simulink model "IonSatSimulationE"  (R2020b)
settings: Solver=ode3  StartTime=0.0  StopTime=t_sim  FixedStep=TimeStep  MaxStep=30  MinStep=.1  RelTol=1e-3
model workspace (MAT data in the model file):
  repartition_matrix = Simulink.Parameter
  repartition_matrix.DataType = 'auto'
  repartition_matrix.Complexity = 'real'
  repartition_matrix.Dimensions = [0 0]
  wheel_number = Simulink.Parameter
  wheel_number.Value = 3
  wheel_number.DataType = 'auto'
  wheel_number.Complexity = 'real'
  wheel_number.Dimensions = [1 1]
values from neighbouring files (symbols this model uses):
  Use_IGRF = 1    [Full_model_PID_MEKF_Scenario1_Monte_Carlo.m]    (also in Full_model_PID_MEKF_Scenario3_Monte_Carlo.m; Full_model_PID_UKF_Scenario1_Monte_Carlo.m; Full_model_PID_UKF_Scenario2_Monte_Carlo.m; Full_model_PID_UKF_Scenario3_Monte_Carlo.m)
  Use_IGRF_KF = 1    [Full_model_PID_MEKF_Scenario1_Monte_Carlo.m]    (also in Full_model_PID_MEKF_Scenario3_Monte_Carlo.m; Full_model_PID_UKF_Scenario1_Monte_Carlo.m; Full_model_PID_UKF_Scenario2_Monte_Carlo.m; Full_model_PID_UKF_Scenario3_Monte_Carlo.m)
undefined symbols (not defined in the file or in its folder): att, date, deg, DiscIntNeverNeededParam, IonSataero, km, m, orbit, rad, s, sat
libraries: aerolibutil x28, vrlib x20, aerolibconvert2 x13, dspmathops x13, sharedtransform x12, simulink x9, DipoleModel x3, aerolibobsolete x3, sharedutil x3, simulink_extras x2, aerolibcelestial x2, dspstat3 x1
(part 1 of 4)
settings Model: SnapshotBufferSize=100  OrderedModelArguments=off  Creator=robin  LastModifiedBy=kang Shinok
settings SolverCC: InitialStep=.5  MaxConsecutiveMinStep=2
settings DataIOCC: SaveFormat=StructureWithTime  SaveOutput=off  SignalLogging=off  DSMLogging=off  SaveTime=off
settings OptimizationCC: DefaultParameterBehavior=Inlined  UseDivisionForNetSlopeComputation=on  GainParamInheritBuiltInType=on  UseFloatMulNetSlope=on  InlineInvariantSignals=on  PassReuseOutputArgsAs=Individual arguments  ZeroExternalMemoryAtStartup=off  ZeroInternalMemoryAtStartup=off  NoFixptDivByZeroProtection=on  EfficientFloat2IntCast=on  LifeSpan=1  OptimizeBlockOrder=speed  DifferentSizesBufferReuse=on  EfficientTunableParamExpr=on
settings DebuggingCC: ParameterTunabilityLossMsg=error
settings HardwareCC: ProdBitPerInt=16  ProdBitPerPointer=8  ProdBitPerSizeT=24  ProdBitPerPtrDiffT=24  ProdLargestAtomicFloat=None  ProdWordSize=8  ProdLongLongMode=on  ProdHWDeviceType=Microchip->PIC18
settings SFSimCC: MATLABDynamicMemAlloc=off  CustomCodeUndefinedFunction=UseInterfaceOnly
settings RTWCC: Description=Embedded Coder  SystemTargetFile=ert.tlc  TemplateMakefile=ert_default_tmf  GenerateReport=on  IncludeHyperlinkInReport=on  LaunchReport=on  GenerateTraceInfo=on  GenerateTraceReport=on  GenerateTraceReportSl=on  GenerateTraceReportSf=on  GenerateTraceReportEml=on  GenerateCodeMetricsReport=on
settings CodeAppCC: ForceParamTrailComments=on  IgnoreCustomStorageClasses=off  OperatorAnnotations=on  SimulinkDataObjDesc=on  SFDataObjDesc=on  CustomSymbolStrGlobalVar=rt$N$M  CustomSymbolStrType=$N$M  CustomSymbolStrFcn=$N$M$F  CustomSymbolStrMacro=$N$M  InsertBlockDesc=on
settings ERTTargetCC: TargetLangStandard=C99 (ISO)  GenerateSampleERTMain=on  IncludeMdlTerminateFcn=off  CombineSignalStateStructs=on  SupportAbsoluteTime=off  SupportComplex=off  SupportContinuousTime=on  SupportNonInlinedSFcns=on  InlinedParameterPlacement=NonHierarchical  ERTCustomFileTemplate=example_file_process.tlc  ERTFilePackagingFormat=CompactWithDataFile

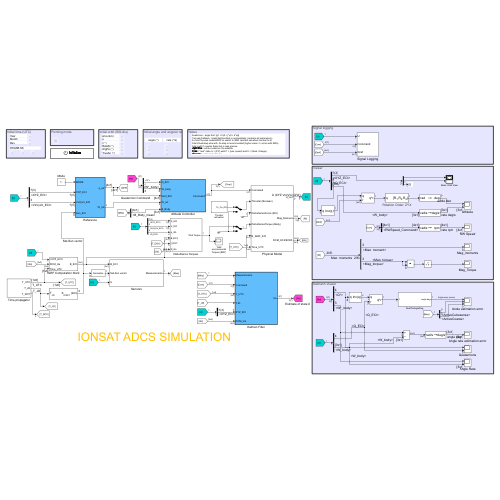
[thumbnail: Simulink's stored preview of the top-level diagram]
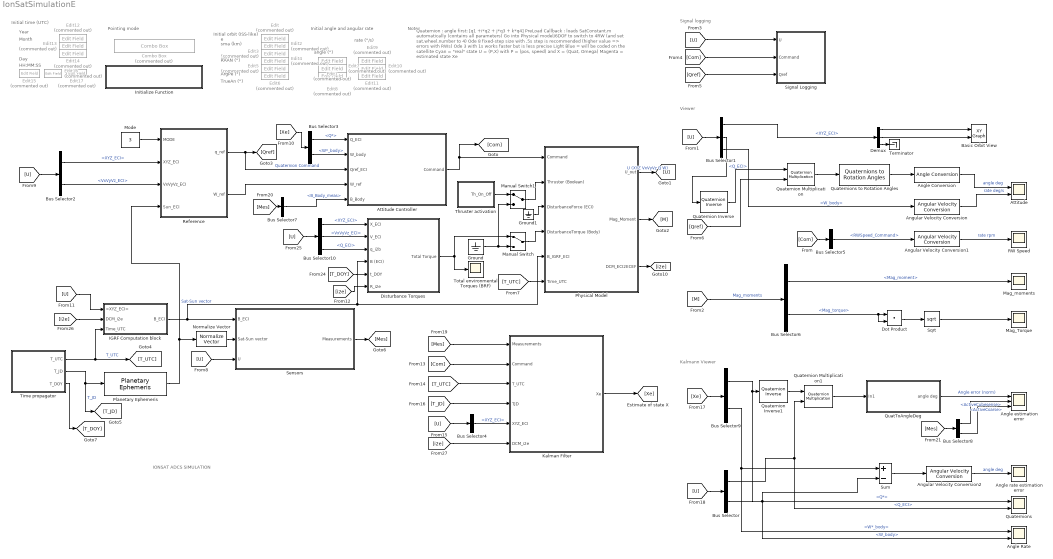
== system IonSatSimulationE ==
  note: Kalmann Viewer
  note: IONSAT ADCS SIMULATION
  note: Viewer
  note: Pointing mode
  note: Initial orbit (ISS-like)
  note: sma (km)
  note: e
  note: i (°)
  note: RAAN (°)
  note: ArgPe (°)
  note: TrueAn (°)
  note: Initial angle and angular rate
  note: angle (°)
  note: rate (°/s)
  note: Notes
  note: Quaternion : angle first: [q1 +i*q2 + j*q3 + k*q4]
      | PreLoad Callback : loads SatConstant.m automatically (contains all parameters)
      | Go into Physical model/6DOF to switch to 4RW (and set sat.wheel.number to 4)
      | Ode 8 fixed-step size with .5s step is recommended (higher value => errors with RWs)
      | Ode 3 with 1s works faster but is less precise
      | Light Blue = will be coded on the satellite
      | Cyan = "real" state U = (P,X) with P = (pos, speed) and X = (Quat, Omega)
      | Magenta = estimated state Xe
  note: Signal logging
  note: Month
  note: Year
  note: Day
  note: Initial time (UTC)
  note: HH:MM:SS
  Angle Conversion : aerolibconvert2/Angle Conversion  IU=rad  OU=deg
  Angle Rate : Scope  NumInputPorts=2
  Angle estimation error : Scope  NumInputPorts=3
  Angle rate estimation error : Scope
  Angular Velocity Conversion : aerolibconvert2/Angular Velocity Conversion  IU=rad/s  OU=deg/s
  Angular Velocity Conversion1 : aerolibconvert2/Angular Velocity Conversion  IU=rad/s  OU=rpm
  Angular Velocity Conversion2 : aerolibconvert2/Angular Velocity Conversion  IU=rad/s  OU=deg/s
  Attitude : Scope  NumInputPorts=2
  Attitude Controller : Subsystem  TreatAsAtomicUnit=on
  Basic Orbit View : simulink/Sinks/XY Graph  xmin=-1  xmax=1  ymin=-1  ymax=1  st=-1
  Bus Selector : BusSelector  OutputSignals=Q_ECI,W_body
  Bus Selector1 : BusSelector  OutputSignals=XYZ_ECI,Q_ECI,W_body
  Bus Selector10 : BusSelector  OutputSignals=XYZ_ECI,VxVyVz_ECI,Q_ECI
  Bus Selector2 : BusSelector  OutputSignals=XYZ_ECI,VxVyVz_ECI
  Bus Selector3 : BusSelector  OutputSignals=Q*,W*_body
  Bus Selector4 : BusSelector  OutputSignals=XYZ_ECI
  Bus Selector5 : BusSelector  OutputSignals=RWSpeed_Command
  Bus Selector6 : BusSelector  OutputSignals=Mag_moment,Mag_torque
  Bus Selector7 : BusSelector  OutputSignals=B_Body_meas
  Bus Selector8 : BusSelector  OutputSignals=ActiveCubesense,ActiveCoarse
  Bus Selector9 : BusSelector  OutputSignals=Q*,W*_body
  Combo Box : ComboBox  Commented=on  LabelPosition=Hide  SelectedLabel=Sun
      settings: Values={{'Nadir', 'Retrograde', 'Drag', 'Sun', 'Sun Aero', 'B-dot', 'Custom Quaternion'}, [1 5 4 3 2 6 7]}
  Demux : Demux  Outputs=3
  Disturbance Torques : Subsystem
  Dot Product : DotProduct  InputSameDT=on  OutDataTypeStr=Inherit: Inherit via internal rule
  Edit{,1..17} (18 alike) : EditField  Commented=on  LabelPosition=Hide  ShowInitialText=on  Alignment=Center
  Ground : Ground
  Ground1 : Ground
  IGRF Computation block : Subsystem
  Initialize Function : Subsystem  TreatAsAtomicUnit=on
  Kalman Filter : Subsystem  TreatAsAtomicUnit=on  SystemSampleTime=1
  Mag_Torque : Scope
  Mag_moments : Scope
  Manual Switch : ManualSwitch
  Manual Switch1 : ManualSwitch
  Mode : Constant  Value=3  OutDataTypeStr=int8
  Normalize Vector : vrlib/Utilities/Normalize Vector  maxzero=0
  Physical Model : Subsystem
      settings: MinAlgLoopOccurrences=on
  Planetary Ephemeris : aerolibcelestial/Planetary Ephemeris  kmflag=km,km/s  epochflag=Julian date  de=DE405  nCenter=Earth  nTarget=Sun  errorflag=Error  velflag=off
      settings: SourceProductBaseCode=AE
  QuatToAngleDeg : Subsystem
  Quaternion Inverse : aerolibutil/Quaternion Inverse
  Quaternion Inverse1 : aerolibutil/Quaternion Inverse
  Quaternion Multiplication : aerolibutil/Quaternion Multiplication
  Quaternion Multiplication1 : aerolibutil/Quaternion Multiplication
  Quaternions : Scope  NumInputPorts=2
  Quaternions to Rotation Angles : sharedtransform/Quaternions to Rotation Angles  rotationOrder=ZYX  aMode=aMode
      settings: SourceProductBaseCode=AE,PW,DR,MT,UV,VE
  RW Speed : Scope
  Reference : Subsystem  TreatAsAtomicUnit=on
  Sensors : Subsystem
  Signal Logging : Subsystem
  Sqrt : Sqrt  SaturateOnIntegerOverflow=on
  Sum : Sum  Inputs=+-
  Terminator : Terminator
  Thruster activation : Subsystem
  Time propagator : Subsystem
  Total environmental Torques (BRF) : Scope
  wires:
  Reference/1(q_ref) -> Attitude Controller/3(Qref_ECI), [Qref]  "Quaternion Command"
  Mode/1 -> Reference/1(MODE)
  Bus Selector2/2 -> Reference/3(VxVyVz_ECI)  "<VxVyVz_ECI>"
  Physical Model/1(U_out) -> [U]  "U (XYZ VxVyVz Q W)"
  Attitude Controller/1(Command) -> Physical Model/1(Command), [Com]
  Angle Conversion/1 -> Attitude/1  "angle deg"
  Demux/3 -> Terminator/1
  Demux/2 -> Basic Orbit View/2
  Angular Velocity Conversion/1 -> Attitude/2  "rate deg/s"
  Bus Selector1/1 -> Demux/1  "<XYZ_ECI>"
  Quaternion Multiplication/1 -> Quaternions to Rotation Angles/1
  Demux/1 -> Basic Orbit View/1
  Bus Selector1/3 -> Angular Velocity Conversion/1  "<W_body>"
  Quaternions to Rotation Angles/1 -> Angle Conversion/1
  Angular Velocity Conversion1/1 -> RW Speed/1  "rate rpm"
  [Com] -> Bus Selector5/1
  [U] -> Bus Selector1/1
  Bus Selector2/1 -> Reference/2(XYZ_ECI)  "<XYZ_ECI>"
  Bus Selector3/2 -> Attitude Controller/2(W_body)  "<W*_body>"
  Planetary Ephemeris/1 -> Reference/4(Sun_ECI), Normalize Vector/1  "Sat-Sun vector"
  [U] -> Signal Logging/1(U)
  [Com] -> Signal Logging/2(Command)
  [Qref] -> Signal Logging/3(Qref)
  [Qref] -> Quaternion Multiplication/2
  Quaternion Inverse/1 -> Quaternion Multiplication/1
  Bus Selector1/2 -> Quaternion Inverse/1  "<Q_ECI>"
  Physical Model/2(Mag_Moment) -> [M]
  [M] -> Bus Selector6/1  "Mag_moments"
  Time propagator/1(T_UTC) -> IGRF Computation block/3("Time_UTC "), [T_UTC]  "T_UTC"
  Time propagator/2(T_JD) -> [T_JD], Planetary Ephemeris/1  "T_JD"
  [U] -> Bus Selector2/1
  [Xe] -> Bus Selector3/1
  [U] -> IGRF Computation block/1(<XYZ_ECI>)
  Kalman Filter/1(Xe) -> [Xe]
  [Com] -> Kalman Filter/2(Command)
  [T_UTC] -> Kalman Filter/3(T_UTC)
  [U] -> Bus Selector4/1
  Bus Selector4/1 -> Kalman Filter/5(XYZ_ECI)  "<XYZ_ECI>"
  [T_JD] -> Kalman Filter/4(TJD)
  [Xe] -> Bus Selector9/1
  [U] -> Bus Selector/1
  Bus Selector9/2 -> Angle Rate/1, Sum/1  "<W*_body>"
  Bus Selector/2 -> Sum/2, Angle Rate/2  "<W_body>"
  Sum/1 -> Angular Velocity Conversion2/1
  Bus Selector9/1 -> Quaternions/1, Quaternion Inverse1/1  "<Q*>"
  Quaternion Inverse1/1 -> Quaternion Multiplication1/1
  Bus Selector/1 -> Quaternions/2, Quaternion Multiplication1/2  "<Q_ECI>"
  Angular Velocity Conversion2/1 -> Angle rate estimation error/1  "angle deg"
  Bus Selector5/1 -> Angular Velocity Conversion1/1  "<RWSpeed_Command>"
  Bus Selector6/1 -> Mag_moments/1  "<Mag_moment>"
  Bus Selector6/2 -> Dot Product/2, Dot Product/1  "<Mag_torque>"
  Dot Product/1 -> Sqrt/1
  Sqrt/1 -> Mag_Torque/1
  Bus Selector7/1 -> Attitude Controller/5(B_Body)  "<B_Body_meas>"
  [U] -> Sensors/3(U)
  Sensors/1(Measurements) -> [Mes]
  [Mes] -> Kalman Filter/1(Measurements)
  [Mes] -> Bus Selector7/1
  [Mes] -> Bus Selector8/1
  Bus Selector8/1 -> Angle estimation error/2  "<ActiveCubesense>"
  Bus Selector8/2 -> Angle estimation error/3  "<ActiveCoarse>"
  Quaternion Multiplication1/1 -> QuatToAngleDeg/1(In1)
  QuatToAngleDeg/1(angle deg) -> Angle estimation error/1  "Angle error (norm)"
  [U] -> Bus Selector10/1
  Bus Selector10/3 -> Disturbance Torques/3(q_i2b)  "<Q_ECI>"
  Bus Selector10/1 -> Disturbance Torques/1(X_ECI)  "<XYZ_ECI>"
  Bus Selector3/1 -> Attitude Controller/1(Q_ECI)  "<Q*>"
  Bus Selector10/2 -> Disturbance Torques/2(V_ECI)  "<VxVyVz_ECI>"
  Time propagator/3(T_DOY) -> [T_DOY]
  [T_DOY] -> Disturbance Torques/5(t_DOY)
  [i2e] -> IGRF Computation block/2("DCM_i2e ")
  IGRF Computation block/1(B_ECI) -> Sensors/1(B_ECI), Physical Model/5(B_IGRF_ECI), Disturbance Torques/4(B (ECI))
  [i2e] -> Kalman Filter/6("DCM_i2e ")
  Normalize Vector/1 -> Sensors/2(Sat-Sun vector)
  [i2e] -> Disturbance Torques/6(R_i2e)
  Ground/1 -> Manual Switch/2, Manual Switch1/2
  Manual Switch1/1 -> Physical Model/2(Thruster (Boolean))
  Thruster activation/1(Th_On_Off) -> Manual Switch1/1
  Disturbance Torques/1("Total Torque ") -> Manual Switch/1, Total environmental Torques (BRF)/1
  Manual Switch/1 -> Physical Model/4(DisturbanceTorque (Body))
  [T_UTC] -> Physical Model/6(Time_UTC)
  Physical Model/3(DCM_ECI2ECEF) -> [i2e]
  Ground1/1 -> Physical Model/3(DisturbanceForce (ECI))
  Reference/2(W_ref) -> Attitude Controller/4(W_ref)

== system IonSatSimulationE/Attitude Controller ==
  note: Choix d'un contrôleur PID : plus simple et robuste qu'un LQR/SliddingSurface ou autre
  note: Runs as fast as possible
  note: Runs at 1Hz
  Q_ECI : Inport
  W_body : Inport  Port=2
  Qref_ECI : Inport  Port=3
  W_ref : Inport  Port=4
  B_Body : Inport  Port=5
  Abs : Abs
  B-dot choice1 : Subsystem
  B-dot choice2 : Subsystem
  B-dot command : Subsystem  TreatAsAtomicUnit=on
  Bus Creator : BusCreator  Inputs=2
  Constant : Constant
  Constant1 : Constant  Value=0
  Ground2 : Ground  Commented=on
  If : If  IfExpression=u1 > 0.068
  If Action Subsystem : Subsystem  TreatAsAtomicUnit=on
  If Action Subsystem1 : Subsystem  TreatAsAtomicUnit=on
  Max of Elements : MinMax  Function=max
  Merge : Merge
  PID (nominal command) : Subsystem  TreatAsAtomicUnit=on  SystemSampleTime=1
  RW4 : Subsystem  Commented=on
  Scope : Scope
  Scope1 : Scope
  Command : Outport  VectorParamsAs1DForOutWhenUnconnected=off
  wires:
  Ground2/1 -> RW4/1(Mc (scalar))
  B_Body/1 -> PID (nominal command)/4(B_IGRF_Body), B-dot command/1(B)
  B-dot choice2/1(output command) -> Bus Creator/2  "Magnetotorquer_Command"
  B-dot choice1/1(output command) -> Bus Creator/1  "RWSpeed_Command"
  B-dot command/2(Wheel command (0)) -> B-dot choice1/2(Command (B-dot))
  B-dot command/1(Magnetic moment (B-dot)) -> B-dot choice2/2(Command (B-dot))
  Q_ECI/1 -> PID (nominal command)/1(Q_ECI)
  Qref_ECI/1 -> PID (nominal command)/2(Qref_ECI)
  PID (nominal command)/1(RW Command) -> B-dot choice1/1(" command (normal)")
  PID (nominal command)/2(Mag Command) -> B-dot choice2/1(" command (normal)")
  Bus Creator/1 -> Command/1
  Abs/1 -> Max of Elements/1
  If/1 -> If Action Subsystem/Action
  If Action Subsystem1/1(Out1) -> Merge/2
  Max of Elements/1 -> Scope1/1, If/1
  If/2 -> If Action Subsystem1/Action
  If Action Subsystem/1(Out1) -> Merge/1
  Constant/1 -> If Action Subsystem/1(In1)
  Merge/1 -> PID (nominal command)/6(No wheels use), Scope/1, B-dot choice2/3(B_dot mode (0/1)), B-dot choice1/3(B_dot mode (0/1))
  Constant1/1 -> If Action Subsystem1/1(In1)
  W_body/1 -> PID (nominal command)/3(W_Body), Abs/1
  W_ref/1 -> PID (nominal command)/5(W_ref)

== system IonSatSimulationE/Disturbance Torques ==
  X_ECI : Inport
  V_ECI : Inport  Port=2
  q_i2b : Inport  Port=3
  B (ECI) : Inport  Port=4
  t_DOY : Inport  Port=5
  R_i2e : Inport  Port=6
  3 dist torques : Scope  NumInputPorts=3
  Add1 : Sum  Inputs=+++
  Aerodynamic Model : Subsystem
  Gravity Gradient Model : Subsystem
  Ground : Ground
  Ground1 : Ground
  Ground2 : Ground
  Magnetic Torque Model : Subsystem
  Manual Switch : ManualSwitch
  Manual Switch1 : ManualSwitch
  Manual Switch2 : ManualSwitch
  Quaternions to Direction Cosine Matrix : sharedtransform/Quaternions to  Direction Cosine Matrix  aMode=aMode
      settings: SourceProductBaseCode=AE,PW,DR,MT,UV,VE
  Total Torque : Scope
  "Total Torque " : Outport
  wires:
  Add1/1 -> Total Torque/1, "Total Torque "/1
  V_ECI/1 -> Aerodynamic Model/1(Velocity  (V) [m/s])
  X_ECI/1 -> Aerodynamic Model/2(Position (X) [m]), Gravity Gradient Model/1("Position (X) [m] ")
  Manual Switch/1 -> 3 dist torques/1, Add1/1  "Aero Torque"
  Manual Switch2/1 -> Add1/3, 3 dist torques/3  "GG Torque"
  B (ECI)/1 -> Magnetic Torque Model/1(B (ECI))
  Manual Switch1/1 -> Add1/2, 3 dist torques/2  "Magnetic Torque"
  q_i2b/1 -> Quaternions to Direction Cosine Matrix/1
  Quaternions to Direction Cosine Matrix/1 -> Gravity Gradient Model/2(Attitude (DCMi2b)), Magnetic Torque Model/2(Attitude (DCMi2b)), Aerodynamic Model/3(Attitude (DCM_i2b))  "i2b"
  R_i2e/1 -> Aerodynamic Model/5(DCM_i2e)
  t_DOY/1 -> Aerodynamic Model/4(DOY)
  Ground/1 -> Manual Switch/2
  Aerodynamic Model/1(Aero. Torque [N.m]) -> Manual Switch/1  "Aero Torque"
  Magnetic Torque Model/1(MagneticTorque (N.m)) -> Manual Switch1/1  "Magnetic Torque"
  Ground1/1 -> Manual Switch1/2
  Ground2/1 -> Manual Switch2/2
  Gravity Gradient Model/1(Gravity Gradient [N.m]) -> Manual Switch2/1  "GG Torque"

== system IonSatSimulationE/IGRF Computation block ==
  <XYZ_ECI> : Inport
  "DCM_i2e " : Inport  Port=2
  "Time_UTC " : Inport  Port=3
  Bus Creator : BusCreator  Inputs=5
  Bus Selector4 : BusSelector  OutputSignals=XYZ_ECI
  Demux : Demux  Outputs=2
  ECI To LLA : MATLAB Function  TreatAsAtomicUnit=on
  Obtain B_ECI : Subsystem
  Product : Product  Multiplication=Matrix(*)
  Reshape : Reshape  OutputDimensionality=Row vector (2-D)
  Terminator : Terminator
  B_ECI : Outport  VectorParamsAs1DForOutWhenUnconnected=off
  wires:
  ECI To LLA/3(long) -> Bus Creator/3
  ECI To LLA/2(lat) -> Bus Creator/2
  ECI To LLA/1(h) -> Bus Creator/1
  Demux/1 -> Bus Creator/4
  Demux/2 -> Terminator/1
  "DCM_i2e "/1 -> Product/2, Bus Creator/5  "DCM_i2e"
  <XYZ_ECI>/1 -> Bus Selector4/1
  Reshape/1 -> Product/1
  Product/1 -> ECI To LLA/1(X_ECEF)
  Bus Selector4/1 -> Reshape/1  "<XYZ_ECI>"
  Bus Creator/1 -> Obtain B_ECI/1(In1)
  Obtain B_ECI/1(Out1) -> B_ECI/1
  "Time_UTC "/1 -> Demux/1

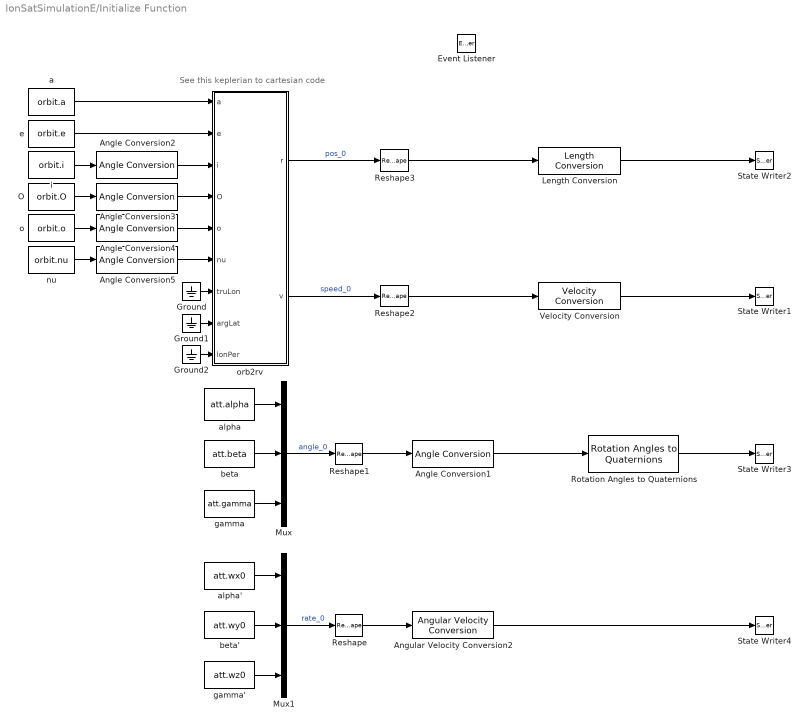
== system IonSatSimulationE/Initialize Function ==
  note: See this keplerian to cartesian code
  Angle Conversion{1..5} (5 alike) : aerolibconvert2/Angle Conversion  IU=deg  OU=rad
  Angular Velocity Conversion2 : aerolibconvert2/Angular Velocity Conversion  IU=deg/s  OU=rad/s
  Event Listener : EventListener  DisableCoverage=on  EventName=reset
  Ground : Ground
  Ground1 : Ground
  Ground2 : Ground
  Length Conversion : aerolibconvert2/Length Conversion  IU=km  OU=m
  Mux : Mux  Inputs=3
  Mux1 : Mux  Inputs=3
  O : Constant  Value=orbit.O
  Reshape{,1..3} (4 alike) : Reshape  OutputDimensionality=Column vector (2-D)
  Rotation Angles to Quaternions : sharedtransform/Rotation Angles to Quaternions  rotationOrder=ZYX  aMode=aMode
      settings: SourceProductBaseCode=AE,PW,DR,MT,UV,VE
  State Writer1 : StateWriter  StateOwnerBlock=../../Physical Model/6DOF in ECI frame/Integrator_speed
  State Writer2 : StateWriter  StateOwnerBlock=../../Physical Model/6DOF in ECI frame/Integrator_pos
  State Writer3 : StateWriter  StateOwnerBlock=../../Physical Model/6DOF in ECI frame/Compute Q_ECI/Integrator_quat
  State Writer4 : StateWriter  StateOwnerBlock=../../Physical Model/6DOF in ECI frame/Integrator_rate
  Velocity Conversion : aerolibconvert2/Velocity Conversion  IU=km/s  OU=m/s
  a : Constant  Value=orbit.a
  alpha : Constant  Value=att.alpha
  alpha' : Constant  Value=att.wx0
  beta : Constant  Value=att.beta
  beta' : Constant  Value=att.wy0
  e : Constant  Value=orbit.e
  gamma : Constant  Value=att.gamma
  gamma' : Constant  Value=att.wz0
  i : Constant  Value=orbit.i
  nu : Constant  Value=orbit.nu
  o : Constant  Value=orbit.o
  orb2rv : MATLAB Function  TreatAsAtomicUnit=on
  wires:
  Angular Velocity Conversion2/1 -> State Writer4/1
  Angle Conversion1/1 -> Rotation Angles to Quaternions/1
  orb2rv/1(r) -> Reshape3/1  "pos_0"
  Mux1/1 -> Reshape/1  "rate_0"
  Mux/1 -> Reshape1/1  "angle_0"
  orb2rv/2(v) -> Reshape2/1  "speed_0"
  Rotation Angles to Quaternions/1 -> State Writer3/1
  Reshape/1 -> Angular Velocity Conversion2/1
  Reshape1/1 -> Angle Conversion1/1
  Reshape2/1 -> Velocity Conversion/1
  Reshape3/1 -> Length Conversion/1
  a/1 -> orb2rv/1(a)
  e/1 -> orb2rv/2(e)
  i/1 -> Angle Conversion2/1
  O/1 -> Angle Conversion3/1
  o/1 -> Angle Conversion4/1
  nu/1 -> Angle Conversion5/1
  Angle Conversion2/1 -> orb2rv/3(i)
  Angle Conversion3/1 -> orb2rv/4(O)
  Angle Conversion4/1 -> orb2rv/5(o)
  Angle Conversion5/1 -> orb2rv/6(nu)
  Ground/1 -> orb2rv/7(truLon)
  Ground1/1 -> orb2rv/8(argLat)
  Ground2/1 -> orb2rv/9(lonPer)
  Length Conversion/1 -> State Writer2/1
  Velocity Conversion/1 -> State Writer1/1
  alpha/1 -> Mux/1
  beta/1 -> Mux/2
  gamma/1 -> Mux/3
  alpha'/1 -> Mux1/1
  gamma'/1 -> Mux1/3
  beta'/1 -> Mux1/2

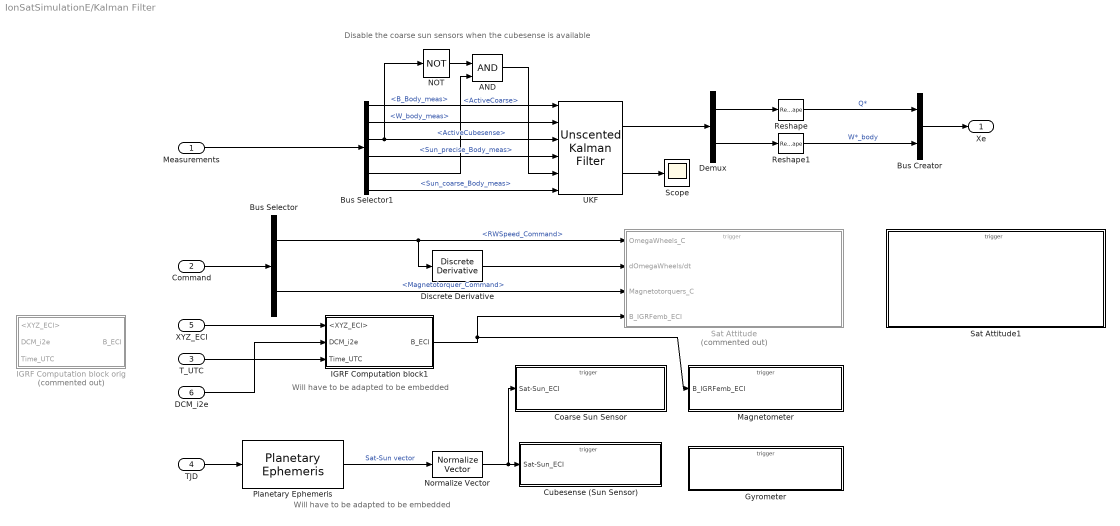
== system IonSatSimulationE/Kalman Filter ==
  note: Disable the coarse sun sensors when the cubesense is available
  note: Will have to be adapted to be embedded
  note: Will have to be adapted to be embedded
  Measurements : Inport
  Command : Inport  Port=2
  T_UTC : Inport  Port=3
  TJD : Inport  Port=4
  XYZ_ECI : Inport  Port=5
  "DCM_i2e " : Inport  Port=6
  AND : Logic  IconShape=distinctive  AllPortsSameDT=off  OutDataTypeStr=boolean
  Bus Creator : BusCreator  Inputs=2
  Bus Selector : BusSelector  OutputSignals=RWSpeed_Command,Magnetotorquer_Command
  Bus Selector1 : BusSelector  OutputSignals=B_Body_meas,W_body_meas,ActiveCubesense,Sun_precise_Body_meas,ActiveCoarse,Sun_coarse_Body_meas
  Coarse Sun Sensor : Subsystem  TreatAsAtomicUnit=on
  Cubesense (Sun Sensor) : Subsystem  TreatAsAtomicUnit=on
  Demux : Demux  Outputs=2
  Discrete Derivative : simulink/Discrete/Discrete Derivative  gainval=1.0  ICPrevScaledInput=0.0  OutMin=[]  OutMax=[]  OutDataType=fixdt(1, 16)  OutScaling=2^-10  DoSatur=off
  Gyrometer : Subsystem  TreatAsAtomicUnit=on
  IGRF Computation block orig : Subsystem  Commented=on
  IGRF Computation block1 : Subsystem
  Magnetometer : Subsystem  TreatAsAtomicUnit=on
  NOT : Logic  Operator=NOT  IconShape=distinctive  AllPortsSameDT=off  OutDataTypeStr=boolean
  Normalize Vector : vrlib/Utilities/Normalize Vector  maxzero=0
  Planetary Ephemeris : aerolibcelestial/Planetary Ephemeris  kmflag=km,km/s  epochflag=Julian date  de=DE405  nCenter=Earth  nTarget=Sun  errorflag=Error  velflag=off
      settings: SourceProductBaseCode=AE
  Reshape : Reshape  OutputDimensionality=Customize  OutputDimensions=[4]
  Reshape1 : Reshape  OutputDimensionality=Customize  OutputDimensions=[3]
  Sat Attitude : Subsystem  Commented=on  TreatAsAtomicUnit=on
  Sat Attitude1 : Subsystem  TreatAsAtomicUnit=on
  Scope : Scope
  UKF : sharedTrackingLibrary/Unscented Kalman Filter  StateTransitionFcn=SatAttitude  HasAdditiveProcessNoise=Additive  ProcessNoise=5e-7  HasTimeVaryingProcessNoise=off  HasStateTransitionFcnExtraArgument=0  InitialState=[1 0 0 0 0 0 0]  InitialStateCovariance=1e-7  Alpha=8e-2  Beta=2  Kappa=0  MeasurementFcn1=MagMeasure  HasMeasurementEnablePort1=off  HasAdditiveMeasurementNoise1=Additive  MeasurementNoise1=sat.sensors.mag_sigma*sat.sensors.mag_sigma*ones(3,1)  HasTimeVaryingMeasurementNoise1=off  HasMeasurementFcnExtraArgument1=0  MeasurementFcn2=GyroMeasure  HasMeasurementEnablePort2=off  HasAdditiveMeasurementNoise2=Additive  MeasurementNoise2=sat.sensors.gyro_sigma*sat.sensors.gyro_sigma*ones(3,1)  HasTimeVaryingMeasurementNoise2=off  HasMeasurementFcnExtraArgument2=0  MeasurementFcn3=SunMeasure  HasMeasurementEnablePort3=on  HasAdditiveMeasurementNoise3=Additive  MeasurementNoise3=sat.sensors.sun_sigma*sat.sensors.sun_sigma*ones(3,1)  HasTimeVaryingMeasurementNoise3=off  HasMeasurementFcnExtraArgument3=0  MeasurementFcn4=SunMeasureCoarse  HasMeasurementEnablePort4=on  HasAdditiveMeasurementNoise4=Additive  MeasurementNoise4=sat.sensors.sun_coarse_sigma*sat.sensors.sun_coarse_sigma*ones(3,1)  HasTimeVaryingMeasurementNoise4=off  HasMeasurementFcnExtraArgument4=0  MeasurementFcn5=myMeasurementFcn  HasMeasurementEnablePort5=off  HasAdditiveMeasurementNoise5=Additive  MeasurementNoise5=1  HasTimeVaryingMeasurementNoise5=off  HasMeasurementFcnExtraArgument5=0  EnableMultirate=off  StateTransitionFcnSampleTime=1  MeasurementFcn1SampleTime=1  MeasurementFcn2SampleTime=1  MeasurementFcn3SampleTime=1  MeasurementFcn4SampleTime=1  MeasurementFcn5SampleTime=1  UseCurrentEstimator=on  OutputStateCovariance=on  DataType=double  SampleTime=1  NumberOfMeasurements=4
      settings: SourceProductBaseCode=AE,PW,CT,DR,TF,ID,LP,NV,AR,RO,RR,UV,VE
  Xe : Outport  VectorParamsAs1DForOutWhenUnconnected=off
  wires:
  Measurements/1 -> Bus Selector1/1
  UKF/1 -> Demux/1
  XYZ_ECI/1 -> IGRF Computation block1/1(<XYZ_ECI>)
  T_UTC/1 -> IGRF Computation block1/3("Time_UTC ")
  IGRF Computation block1/1(B_ECI) -> Sat Attitude/4(B_IGRFemb_ECI), Magnetometer/1(B_IGRFemb_ECI)
  Command/1 -> Bus Selector/1
  Bus Selector/1 -> Discrete Derivative/1, Sat Attitude/1(OmegaWheels_C)  "<RWSpeed_Command>"
  Bus Selector/2 -> Sat Attitude/3(Magnetotorquers_C)  "<Magnetotorquer_Command>"
  TJD/1 -> Planetary Ephemeris/1
  Bus Selector1/1 -> UKF/1  "<B_Body_meas>"
  Bus Selector1/2 -> UKF/2  "<W_body_meas>"
  Bus Selector1/6 -> UKF/6  "<Sun_coarse_Body_meas>"
  Planetary Ephemeris/1 -> Normalize Vector/1  "Sat-Sun vector"
  Discrete Derivative/1 -> Sat Attitude/2(dOmegaWheels/dt)
  Bus Selector1/3 -> UKF/3, NOT/1  "<ActiveCubesense>"
  Bus Selector1/4 -> UKF/4  "<Sun_precise_Body_meas>"
  Bus Selector1/5 -> AND/2  "<ActiveCoarse>"
  NOT/1 -> AND/1
  AND/1 -> UKF/5
  UKF/2 -> Scope/1
  Bus Creator/1 -> Xe/1
  Demux/1 -> Reshape/1
  Demux/2 -> Reshape1/1
  Reshape/1 -> Bus Creator/1  "Q*"
  Reshape1/1 -> Bus Creator/2  "W*_body"
  "DCM_i2e "/1 -> IGRF Computation block1/2("DCM_i2e ")
  Normalize Vector/1 -> Coarse Sun Sensor/1(Sat-Sun_ECI), Cubesense (Sun Sensor)/1(Sat-Sun_ECI)

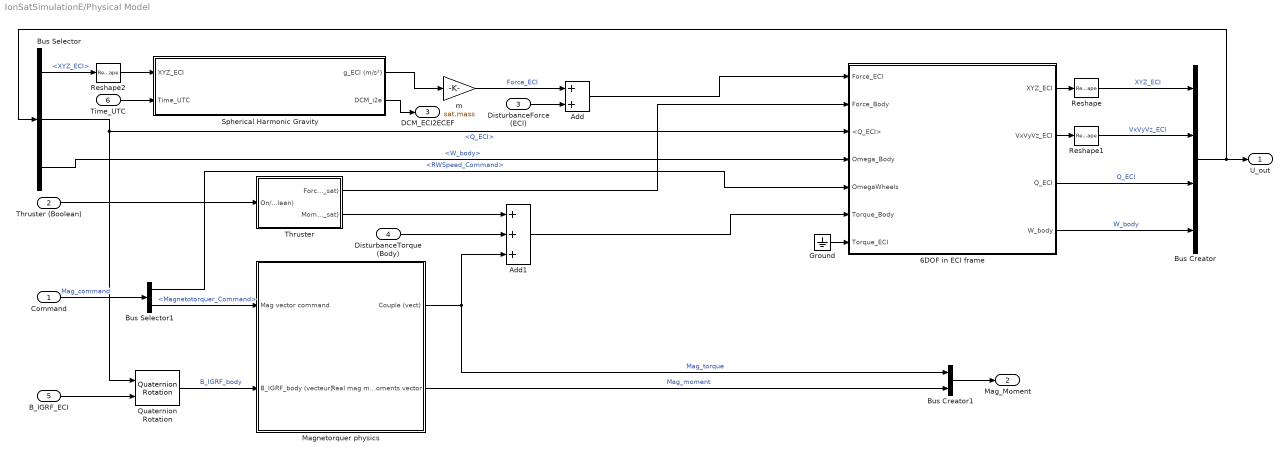
== system IonSatSimulationE/Physical Model ==
  Command : Inport
  Thruster (Boolean) : Inport  Port=2
  DisturbanceForce (ECI) : Inport  Port=3
  DisturbanceTorque (Body) : Inport  Port=4
  B_IGRF_ECI : Inport  Port=5
  Time_UTC : Inport  Port=6
  6DOF in ECI frame : Subsystem
  Add : Sum
  Add1 : Sum  Inputs=+++
  Bus Creator : BusCreator  Inputs=4
  Bus Creator1 : BusCreator  Inputs=2
  Bus Selector : BusSelector  OutputSignals=XYZ_ECI,Q_ECI,W_body
  Bus Selector1 : BusSelector  OutputSignals=RWSpeed_Command,Magnetotorquer_Command
  Ground : Ground
  Magnetorquer physics : Subsystem
  Quaternion Rotation : aerolibutil/Quaternion Rotation
  Reshape : Reshape
  Reshape1 : Reshape
  Reshape2 : Reshape  OutputDimensionality=Column vector (2-D)
  Spherical Harmonic Gravity : Subsystem  TreatAsAtomicUnit=on  SystemSampleTime=1
  Thruster : Subsystem
  m : Gain  Gain=sat.mass
  U_out : Outport  VectorParamsAs1DForOutWhenUnconnected=off
  Mag_Moment : Outport  Port=2  VectorParamsAs1DForOutWhenUnconnected=off
  DCM_ECI2ECEF : Outport  Port=3
  wires:
  Bus Selector/1 -> Reshape2/1  "<XYZ_ECI>"
  Spherical Harmonic Gravity/1(g_ECI (m/s²)) -> m/1
  Thruster (Boolean)/1 -> Thruster/1(On/Off (Boolean))
  Bus Creator/1 -> Bus Selector/1, U_out/1
  Bus Selector/2 -> 6DOF in ECI frame/3(<Q_ECI>), Quaternion Rotation/1  "<Q_ECI>"
  6DOF in ECI frame/3(Q_ECI) -> Bus Creator/3  "Q_ECI"
  6DOF in ECI frame/1(XYZ_ECI) -> Reshape/1
  6DOF in ECI frame/2(VxVyVz_ECI) -> Reshape1/1
  m/1 -> Add/1  "Force_ECI"
  Add/1 -> 6DOF in ECI frame/1(Force_ECI)
  Thruster/1(Force (G_sat)) -> 6DOF in ECI frame/2(Force_Body)
  Bus Selector1/2 -> Magnetorquer physics/1(Mag vector command)  "<Magnetotorquer_Command>"
  Thruster/2(Moment (G_sat)) -> Add1/1
  Add1/1 -> 6DOF in ECI frame/6(Torque_Body)
  DisturbanceForce (ECI)/1 -> Add/2
  DisturbanceTorque (Body)/1 -> Add1/2
  Reshape/1 -> Bus Creator/1  "XYZ_ECI"
  Reshape1/1 -> Bus Creator/2  "VxVyVz_ECI"
  Reshape2/1 -> Spherical Harmonic Gravity/1(XYZ_ECI)
  Bus Selector/3 -> 6DOF in ECI frame/4("Omega_Body ")  "<W_body>"
  Time_UTC/1 -> Spherical Harmonic Gravity/2(Time_UTC)
  B_IGRF_ECI/1 -> Quaternion Rotation/2
  Quaternion Rotation/1 -> Magnetorquer physics/2(B_IGRF_body (vecteur))  "B_IGRF_body"
  Magnetorquer physics/2(Real mag moments vector) -> Bus Creator1/2  "Mag_moment"
  Magnetorquer physics/1(Couple (vect)) -> Add1/3, Bus Creator1/1  "Mag_torque"
  6DOF in ECI frame/4(W_body) -> Bus Creator/4  "W_body"
  Command/1 -> Bus Selector1/1  "Mag_command"
  Bus Selector1/1 -> 6DOF in ECI frame/5(OmegaWheels)  "<RWSpeed_Command>"
  Bus Creator1/1 -> Mag_Moment/1
  Spherical Harmonic Gravity/2(DCM_i2e) -> DCM_ECI2ECEF/1
  Ground/1 -> 6DOF in ECI frame/7(Torque_ECI)

== system IonSatSimulationE/QuatToAngleDeg ==
  In1 : Inport
  Abs : Abs
  Angle Conversion1 : aerolibconvert2/Angle Conversion  IU=rad  OU=deg
  Demux1 : Demux
  Quaternion to axis and angle conversion : MATLABFcn  MATLABFcn=quat2axisangle
  Terminator1 : Terminator
  Terminator2 : Terminator
  Terminator3 : Terminator
  angle deg : Outport  VectorParamsAs1DForOutWhenUnconnected=off
  wires:
  Demux1/2 -> Terminator2/1
  Demux1/4 -> Angle Conversion1/1
  In1/1 -> Quaternion to axis and angle conversion/1
  Demux1/1 -> Terminator1/1
  Demux1/3 -> Terminator3/1
  Quaternion to axis and angle conversion/1 -> Demux1/1
  Abs/1 -> angle deg/1
  Angle Conversion1/1 -> Abs/1  "angle deg"

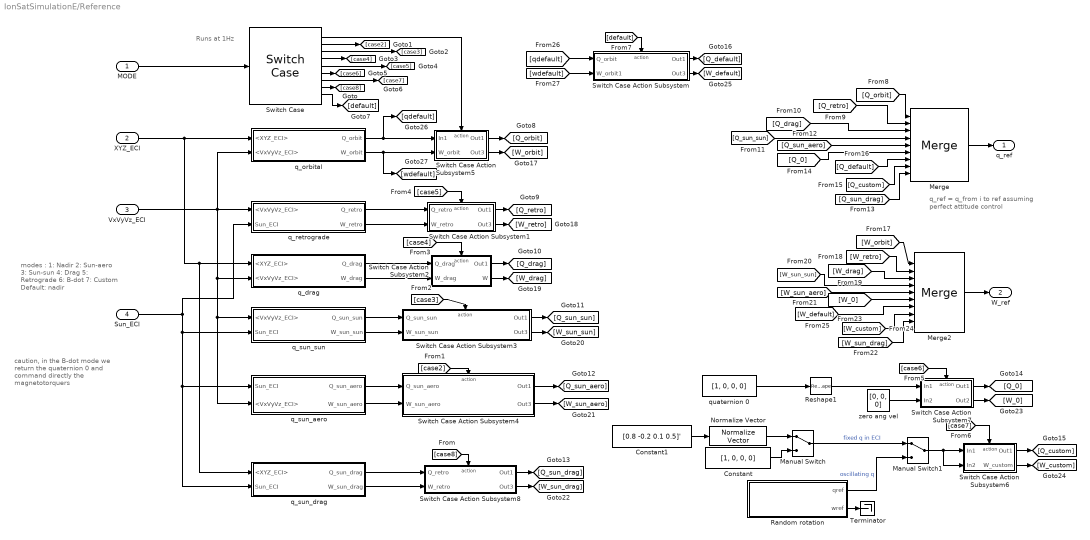
== system IonSatSimulationE/Reference ==
  note: caution, in the B-dot mode we return the quaternion 0 and command directly the magnetotorquers
  note: modes :
      | 1: Nadir
      | 2: Sun-aero
      | 3: Sun-sun
      | 4: Drag
      | 5: Retrograde
      | 6: B-dot
      | 7: Custom
      | Default: nadir
  note: q_ref  = q_from i to ref
      | assuming perfect attitude control
  note: Runs at 1Hz
  MODE : Inport  OutMin=1  OutMax=100  OutDataTypeStr=int8
  XYZ_ECI : Inport  Port=2
  VxVyVz_ECI : Inport  Port=3
  Sun_ECI : Inport  Port=4
  Constant : Constant  Value=[1, 0, 0, 0]
  Constant1 : Constant  Value=[0.8 -0.2 0.1 0.5]'
  Manual Switch : ManualSwitch
  Manual Switch1 : ManualSwitch
  Merge : Merge  Inputs=9
  Merge2 : Merge  Inputs=9
  Normalize Vector : vrlib/Utilities/Normalize Vector  maxzero=0
  Random rotation : Subsystem
  Reshape1 : Reshape  OutputDimensionality=Column vector (2-D)
  Switch Case : SwitchCase  CaseConditions={1, 2, 3, 4, 5, 6, 7, 8}
  Switch Case Action Subsystem : Subsystem  TreatAsAtomicUnit=on
  Switch Case Action Subsystem1 : Subsystem  TreatAsAtomicUnit=on
  Switch Case Action Subsystem2 : Subsystem  TreatAsAtomicUnit=on
  Switch Case Action Subsystem3 : Subsystem  TreatAsAtomicUnit=on
  Switch Case Action Subsystem4 : Subsystem  TreatAsAtomicUnit=on
  Switch Case Action Subsystem5 : Subsystem  TreatAsAtomicUnit=on
  Switch Case Action Subsystem6 : Subsystem  TreatAsAtomicUnit=on
  Switch Case Action Subsystem7 : Subsystem  TreatAsAtomicUnit=on
  Switch Case Action Subsystem8 : Subsystem  TreatAsAtomicUnit=on
  Terminator : Terminator
  q_drag : Subsystem
  q_orbital : Subsystem
  q_retrograde : Subsystem
  q_sun_aero : Subsystem
  q_sun_drag : Subsystem
  q_sun_sun : Subsystem
  quaternion 0 : Constant  Value=[1, 0, 0, 0]
  zero ang vel : Constant  Value=[0, 0, 0]
  q_ref : Outport  VectorParamsAs1DForOutWhenUnconnected=off
  W_ref : Outport  Port=2
  wires:
  quaternion 0/1 -> Reshape1/1
  Reshape1/1 -> Switch Case Action Subsystem7/1(In1)
  Constant/1 -> Manual Switch/2
  Constant1/1 -> Normalize Vector/1
  Normalize Vector/1 -> Manual Switch/1
  zero ang vel/1 -> Switch Case Action Subsystem7/2(In2)
  Manual Switch/1 -> Manual Switch1/1  "fixed q in ECI"
  Random rotation/1(qref) -> Manual Switch1/2  "oscillating q"
  Manual Switch1/1 -> Switch Case Action Subsystem6/2(In2), Switch Case Action Subsystem6/1(In1)
  XYZ_ECI/1 -> q_sun_drag/1(<XYZ_ECI>), q_drag/1(<XYZ_ECI>), q_orbital/1(<XYZ_ECI>)
  [default] -> Switch Case Action Subsystem/Action
  Switch Case/7 -> [case7]
  Switch Case/4 -> [case4]
  Switch Case/5 -> [case5]
  [case3] -> Switch Case Action Subsystem3/Action
  [case5] -> Switch Case Action Subsystem1/Action
  Switch Case/3 -> [case3]
  Switch Case/2 -> [case2]
  q_drag/2(W_drag) -> Switch Case Action Subsystem2/2(W_drag)
  q_sun_drag/2(W_sun_drag) -> Switch Case Action Subsystem8/2(W_retro)
  q_sun_aero/2(W_sun_aero) -> Switch Case Action Subsystem4/2(W_sun_aero)
  Switch Case/1 -> Switch Case Action Subsystem5/Action
  [case8] -> Switch Case Action Subsystem8/Action
  Switch Case/8 -> [case8]
  q_drag/1(Q_drag) -> Switch Case Action Subsystem2/1(Q_drag)
  Switch Case/9 -> [default]
  Sun_ECI/1 -> q_retrograde/2(Sun_ECI), q_sun_drag/2(Sun_ECI), q_sun_aero/1(Sun_ECI), q_sun_sun/2(Sun_ECI)
  q_sun_sun/2(W_sun_sun) -> Switch Case Action Subsystem3/2(W_sun_sun)
  q_retrograde/2(W_retro) -> Switch Case Action Subsystem1/2(W_retro)
  q_sun_sun/1(Q_sun_sun) -> Switch Case Action Subsystem3/1(Q_sun_sun)
  q_sun_aero/1(Q_sun_aero) -> Switch Case Action Subsystem4/1(Q_sun_aero)
  q_sun_drag/1(Q_sun_drag) -> Switch Case Action Subsystem8/1(Q_retro)
  Merge2/1 -> W_ref/1
  [case2] -> Switch Case Action Subsystem4/Action
  [case4] -> Switch Case Action Subsystem2/Action
  q_orbital/1(Q_orbit) -> [qdefault], Switch Case Action Subsystem5/1(In1)
  q_retrograde/1(Q_retro) -> Switch Case Action Subsystem1/1(Q_retro)
  q_orbital/2(W_orbit) -> [wdefault], Switch Case Action Subsystem5/2(W_orbit)
  Switch Case/6 -> [case6]
  VxVyVz_ECI/1 -> q_orbital/2(<VxVyVz_ECI>), q_retrograde/1(<VxVyVz_ECI>), q_drag/2(<VxVyVz_ECI>), q_sun_aero/2(<VxVyVz_ECI>), q_sun_sun/1(<VxVyVz_ECI>)
  Merge/1 -> q_ref/1
  MODE/1 -> Switch Case/1
  Random rotation/2(wref) -> Terminator/1
  [case6] -> Switch Case Action Subsystem7/Action
  [case7] -> Switch Case Action Subsystem6/Action
  Switch Case Action Subsystem5/1(Out1) -> [Q_orbit]
  [Q_orbit] -> Merge/1
  Switch Case Action Subsystem1/1(Out1) -> [Q_retro]
  [Q_retro] -> Merge/2
  Switch Case Action Subsystem2/1(Out1) -> [Q_drag]
  [Q_drag] -> Merge/3
  Switch Case Action Subsystem3/1(Out1) -> [Q_sun_sun]
  [Q_sun_sun] -> Merge/4
  Switch Case Action Subsystem4/1(Out1) -> [Q_sun_aero]
  [Q_sun_aero] -> Merge/5
  Switch Case Action Subsystem8/1(Out1) -> [Q_sun_drag]
  [Q_sun_drag] -> Merge/9
  Switch Case Action Subsystem7/1(Out1) -> [Q_0]
  [Q_0] -> Merge/6
  Switch Case Action Subsystem6/1(Out1) -> [Q_custom]
  [Q_custom] -> Merge/8
  Switch Case Action Subsystem/1(Out1) -> [Q_default]
  [Q_default] -> Merge/7
  Switch Case Action Subsystem5/2(Out3) -> [W_orbit]
  [W_orbit] -> Merge2/1
  Switch Case Action Subsystem1/2(Out3) -> [W_retro]
  [W_retro] -> Merge2/2
  Switch Case Action Subsystem2/2(W) -> [W_drag]
  [W_drag] -> Merge2/3
  Switch Case Action Subsystem3/2(Out3) -> [W_sun_sun]
  [W_sun_sun] -> Merge2/4
  Switch Case Action Subsystem4/2(Out3) -> [W_sun_aero]
  [W_sun_aero] -> Merge2/5
  Switch Case Action Subsystem8/2(Out3) -> [W_sun_drag]
  [W_sun_drag] -> Merge2/9
  Switch Case Action Subsystem7/2(Out2) -> [W_0]
  [W_0] -> Merge2/6
  Switch Case Action Subsystem6/2(W_custom) -> [W_custom]
  [W_custom] -> Merge2/8
  Switch Case Action Subsystem/2(Out3) -> [W_default]
  [W_default] -> Merge2/7
  [qdefault] -> Switch Case Action Subsystem/1(Q_orbit)
  [wdefault] -> Switch Case Action Subsystem/2(W_orbit1)

== system IonSatSimulationE/Sensors ==
  B_ECI : Inport
  Sat-Sun vector : Inport  Port=2
  U : Inport  Port=3
  Bus Creator : BusCreator  Inputs=6
  MEMS Gyro : Subsystem
  Magnetometer : Subsystem
  Sun Sensor (Coarse) : Subsystem
  Sun Sensor (Sun sensor) : Subsystem
  Measurements : Outport  VectorParamsAs1DForOutWhenUnconnected=off
  wires:
  Sat-Sun vector/1 -> Sun Sensor (Coarse)/1(Sat-Sun_ECI), Sun Sensor (Sun sensor)/1(Sat-Sun_ECI)
  MEMS Gyro/1(W_Body_meas) -> Bus Creator/2  "W_body_meas"
  U/1 -> Magnetometer/1(U), MEMS Gyro/1(U), Sun Sensor (Coarse)/2(U), Sun Sensor (Sun sensor)/2(U)
  Magnetometer/1(B_Body_meas) -> Bus Creator/1  "B_Body_meas"
  Sun Sensor (Sun sensor)/1(Sat-Sun_precise_body_meas) -> Bus Creator/3  "Sun_precise_Body_meas"
  Sun Sensor (Coarse)/1(Sat-Sun_coarse_body_meas) -> Bus Creator/5  "Sun_coarse_Body_meas"
  Sun Sensor (Sun sensor)/2(Sensor active (bool)) -> Bus Creator/4  "ActiveCubesense"
  Sun Sensor (Coarse)/2(Sensor active (bool)) -> Bus Creator/6  "ActiveCoarse"
  Bus Creator/1 -> Measurements/1
  B_ECI/1 -> Magnetometer/2(B_IGRF_ECI)

== system IonSatSimulationE/Signal Logging ==
  U : Inport
  Command : Inport  Port=2
  Qref : Inport  Port=3
  Bus Selector : BusSelector  OutputSignals=RWSpeed_Command,Magnetotorquer_Command
  Bus Selector4 : BusSelector  OutputSignals=XYZ_ECI,VxVyVz_ECI,Q_ECI,W_body
  Dot Product : DotProduct  InputSameDT=on  OutDataTypeStr=Inherit: Inherit via internal rule
  Reshape : Reshape
  Reshape1 : Reshape
  Reshape2 : Reshape
  Scope : Scope
  Sqrt : Sqrt  SaturateOnIntegerOverflow=on
  To Workspace : ToWorkspace  VariableName=sat_pos  SaveFormat=Timeseries  SampleTime=1
      settings: Save2DSignal=2-D array (concatenate along first dimension)
  To Workspace1 : ToWorkspace  VariableName=sat_speed  SaveFormat=Timeseries  SampleTime=1
      settings: Save2DSignal=2-D array (concatenate along first dimension)
  To Workspace2 : ToWorkspace  VariableName=sat_Q  SaveFormat=Timeseries  SampleTime=1
      settings: Save2DSignal=2-D array (concatenate along first dimension)
  To Workspace3 : ToWorkspace  VariableName=sat_omega  SaveFormat=Timeseries  SampleTime=1
      settings: Save2DSignal=2-D array (concatenate along first dimension)
  To Workspace4 : ToWorkspace  VariableName=RWSpeed_Command  SaveFormat=Timeseries  SampleTime=1
      settings: Save2DSignal=2-D array (concatenate along first dimension)
  To Workspace5 : ToWorkspace  VariableName=sat_Qc  SaveFormat=Timeseries  SampleTime=1
      settings: Save2DSignal=2-D array (concatenate along first dimension)
  To Workspace6 : ToWorkspace  VariableName=Mag_Command  SaveFormat=Timeseries  SampleTime=1
      settings: Save2DSignal=2-D array (concatenate along first dimension)
  wires:
  Bus Selector4/3 -> To Workspace2/1  "<Q_ECI>"
  Bus Selector4/4 -> To Workspace3/1  "<W_body>"
  U/1 -> Bus Selector4/1
  Bus Selector4/2 -> To Workspace1/1  "<VxVyVz_ECI>"
  Command/1 -> Bus Selector/1
  Bus Selector4/1 -> Dot Product/2, Dot Product/1, To Workspace/1  "<XYZ_ECI>"
  Qref/1 -> Reshape1/1
  Reshape/1 -> To Workspace4/1
  Reshape1/1 -> To Workspace5/1
  Bus Selector/1 -> Reshape/1  "<RWSpeed_Command>"
  Bus Selector/2 -> Reshape2/1  "<Magnetotorquer_Command>"
  Reshape2/1 -> To Workspace6/1
  Dot Product/1 -> Sqrt/1
  Sqrt/1 -> Scope/1

== system IonSatSimulationE/Thruster activation ==
  Clock1 : Clock
  Constant3 : Constant  Value=sat.thruster.duration
  Constant4 : Constant  Value=sat.thruster.firstimpulse
  Constant5 : Constant  Value=sat.thruster.wait
  Constant6 : Constant  Value=sat.thruster.Nfirings
  MATLAB Function : MATLAB Function  TreatAsAtomicUnit=on
  Mux1 : Mux  Inputs=5
  Scope : Scope
  Th_On_Off : Outport  VectorParamsAs1DForOutWhenUnconnected=off
  wires:
  MATLAB Function/1(y) -> Scope/1, Th_On_Off/1
  Clock1/1 -> Mux1/1
  Constant3/1 -> Mux1/2
  Constant4/1 -> Mux1/3
  Constant5/1 -> Mux1/4
  Constant6/1 -> Mux1/5
  Mux1/1 -> MATLAB Function/1(u)

== system IonSatSimulationE/Time propagator ==
  note: Time initialization
  Add : Sum  Inputs=|++
  Clock : Clock
  Constant : Constant  Value=86400
  Day : Constant  Value=date.day
  Divide : Product  Inputs=*/
  HH : Constant  Value=date.hours
  JD to UTC : MATLAB Function  TreatAsAtomicUnit=on
  MATLAB Function : MATLAB Function  TreatAsAtomicUnit=on
  MM : Constant  Value=date.minutes
  Month : Constant  Value=date.month
  Mux : Mux  Inputs=6
  Mux1 : Mux  Inputs=3
  Reshape : Reshape
  SS : Constant  Value=date.seconds
  Signal logging : ToWorkspace  VariableName=T_UTC  SaveFormat=Timeseries  SampleTime=1
      settings: Save2DSignal=2-D array (concatenate along first dimension)
  Signal logging1 : ToWorkspace  VariableName=T_JD  SaveFormat=Timeseries  SampleTime=1
      settings: Save2DSignal=2-D array (concatenate along first dimension)
  UTC to JD : MATLAB Function  TreatAsAtomicUnit=on
  Year : Constant  Value=date.year
  T_UTC : Outport  VectorParamsAs1DForOutWhenUnconnected=off
  T_JD : Outport  Port=2  VectorParamsAs1DForOutWhenUnconnected=off
  T_DOY : Outport  Port=3
  wires:
  UTC to JD/1(JD) -> Add/1  "JD_0"
  Clock/1 -> MATLAB Function/1(t), Divide/1
  Constant/1 -> Divide/2
  JD to UTC/1(Time_UTC) -> T_UTC/1, Reshape/1
  Divide/1 -> Add/2
  Mux/1 -> UTC to JD/1(Time_UTC)
  Day/1 -> Mux/3
  Month/1 -> Mux/2
  Year/1 -> Mux/1
  HH/1 -> Mux/4
  MM/1 -> Mux/5
  SS/1 -> Mux/6
  Reshape/1 -> Signal logging/1
  Add/1 -> Signal logging1/1, T_JD/1, JD to UTC/1(JD)
  MATLAB Function/1(Y) -> Mux1/1
  MATLAB Function/2(DOY) -> Mux1/2
  MATLAB Function/3(S) -> Mux1/3
  Mux1/1 -> T_DOY/1

== system IonSatSimulationE/Attitude Controller/B-dot choice1 ==
  " command (normal)" : Inport
  Command (B-dot) : Inport  Port=2
  B_dot mode (0/1) : Inport  Port=3
  If1 : If
  Merge : Merge
  Switch Case Action Subsystem3 : Subsystem  TreatAsAtomicUnit=on
  Switch Case Action Subsystem4 : Subsystem  TreatAsAtomicUnit=on
  output command : Outport  VectorParamsAs1DForOutWhenUnconnected=off
  wires:
  If1/2 -> Switch Case Action Subsystem4/Action
  If1/1 -> Switch Case Action Subsystem3/Action
  B_dot mode (0/1)/1 -> If1/1
  Command (B-dot)/1 -> Switch Case Action Subsystem3/1(In1)
  Merge/1 -> output command/1
  Switch Case Action Subsystem3/1(Out1) -> Merge/1
  Switch Case Action Subsystem4/1(Out1) -> Merge/2
  " command (normal)"/1 -> Switch Case Action Subsystem4/1(In1)

== system IonSatSimulationE/Attitude Controller/B-dot choice2 ==
  " command (normal)" : Inport
  Command (B-dot) : Inport  Port=2
  B_dot mode (0/1) : Inport  Port=3
  If1 : If
  Merge : Merge
  Switch Case Action Subsystem3 : Subsystem  TreatAsAtomicUnit=on
  Switch Case Action Subsystem4 : Subsystem  TreatAsAtomicUnit=on
  output command : Outport  VectorParamsAs1DForOutWhenUnconnected=off
  wires:
  If1/2 -> Switch Case Action Subsystem4/Action
  If1/1 -> Switch Case Action Subsystem3/Action
  B_dot mode (0/1)/1 -> If1/1
  Command (B-dot)/1 -> Switch Case Action Subsystem3/1(In1)
  Switch Case Action Subsystem3/1(Out1) -> Merge/1
  Switch Case Action Subsystem4/1(Out1) -> Merge/2
  " command (normal)"/1 -> Switch Case Action Subsystem4/1(In1)
  Merge/1 -> output command/1

== system IonSatSimulationE/Attitude Controller/B-dot command ==
  note: ref : OneDrive\IonSat X18\SCAO\Contrôle attitude\Detumbling\Detumbling and Aerostable Control for Cubesats.pdf
      |
      | formulae:
      | $\mathbf{\dot B} \simeq \mathbf{B}\times \mathbf{\dot \theta}$
      | $\mathbf{m} = -c\mathbf{\dot B}$
      |
      | this block does NOT decide if the B-dot mode is relevant or not
      | (it applies it without question on the rotation rate :
      | $\Omega=v/r= \sqrt{\frac{Gm_{earth}}{(h+r_{earth})^{3/2}}} \sim 0.066 °/s$ So the command MUST stop the B-dot mode when the estimated rotation speed is smaller than 0.1 degree per second )
  note: entrée:
      | champ magnétique
      | sortie: moment magnetique de commande et vitesse des roues à réaction (nulle)
  B : Inport
  Discrete Derivative : simulink/Discrete/Discrete Derivative  gainval=1.0  ICPrevScaledInput=0.0  OutMin=[]  OutMax=[]  OutDataType=fixdt(1, 16)  OutScaling=2^-10  DoSatur=off
  Divide1 : Product  Inputs=**
  Reshape2 : Reshape  OutputDimensionality=Column vector (2-D)
  constant c : Constant  Value=-sat.bdot_c
  wheels unused : Constant  Value=[0, 0, 0, 0]
  Magnetic moment (B-dot) : Outport  VectorParamsAs1DForOutWhenUnconnected=off
  Wheel command (0) : Outport  Port=2  VectorParamsAs1DForOutWhenUnconnected=off
  wires:
  constant c/1 -> Divide1/2
  B/1 -> Discrete Derivative/1
  Discrete Derivative/1 -> Divide1/1  "B_point=B^theta_point"
  Divide1/1 -> Magnetic moment (B-dot)/1
  wheels unused/1 -> Reshape2/1
  Reshape2/1 -> Wheel command (0)/1

== system IonSatSimulationE/Attitude Controller/If Action Subsystem ==
  In1 : Inport
  Action Port : ActionPort  ActionPortLabel=if(u1 > 0.068)
  Out1 : Outport  VectorParamsAs1DForOutWhenUnconnected=off
  wires:
  In1/1 -> Out1/1

== system IonSatSimulationE/Attitude Controller/If Action Subsystem1 ==
  In1 : Inport
  Action Port : ActionPort  ActionPortLabel=else
  Out1 : Outport  VectorParamsAs1DForOutWhenUnconnected=off
  wires:
  In1/1 -> Out1/1

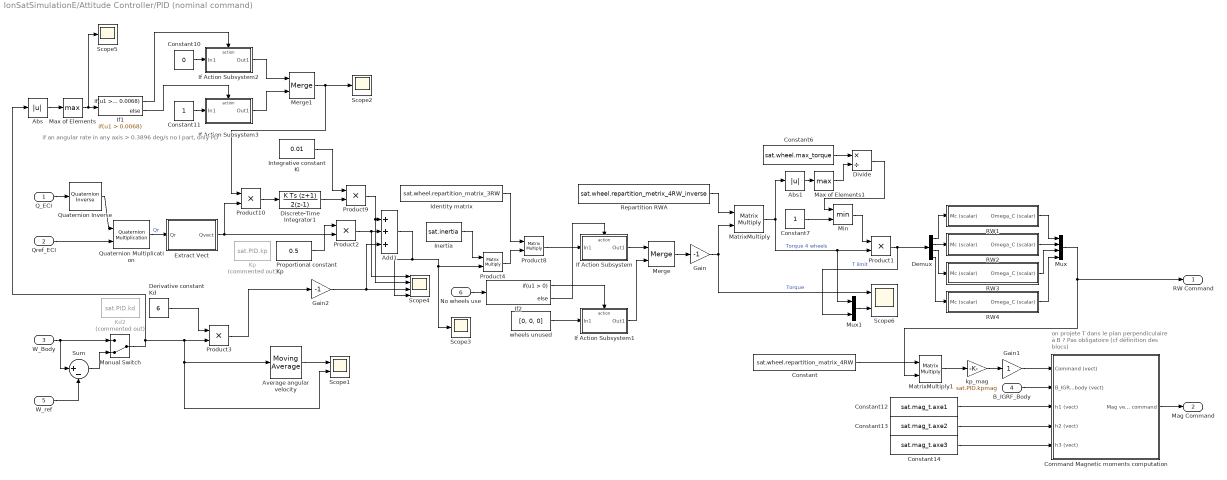
== system IonSatSimulationE/Attitude Controller/PID (nominal command) ==
  note: if an angular rate in any axis > 0.3896 deg/s no I part, only PD
  note: on projete T dans
      | le plan perpendiculaire à B ?
      | Pas obligatoire (cf définition des blocs)
  Q_ECI : Inport
  Qref_ECI : Inport  Port=2
  W_Body : Inport  Port=3
  B_IGRF_Body : Inport  Port=4
  W_ref : Inport  Port=5
  No wheels use : Inport  Port=6
  Abs : Abs
  Abs1 : Abs
  Add1 : Sum  Inputs=+++
  Average angular velocity : dspstat3/Moving Average  Method=Sliding window  ForgettingFactorPort=off  SpecifyWindowLength=on  WindowLength=4  ForgettingFactor=0.9  SimulateUsing=Code generation
  Command Magnetic moments computation : Subsystem
  Constant : Constant  Value=sat.wheel.repartition_matrix_4RW
  Constant10 : Constant  Value=0
  Constant11 : Constant
  Constant12 : Constant  Value=sat.mag_t.axe1
  Constant13 : Constant  Value=sat.mag_t.axe2
  Constant14 : Constant  Value=sat.mag_t.axe3
  Constant6 : Constant  Value=sat.wheel.max_torque
  Constant7 : Constant
  Demux : Demux
  Derivative constant Kd : Constant  Value=6
  Discrete-Time Integrator1 : DiscreteIntegrator  IntegratorMethod=Integration: Trapezoidal  SampleTime=-1  ICPrevOutput=DiscIntNeverNeededParam  ICPrevScaledInput=DiscIntNeverNeededParam
  Divide : Product  Inputs=*/
  Extract Vect : Subsystem
  Gain : Gain  Gain=-1
  Gain1 : Gain
  Gain2 : Gain  Gain=-1
  Identity matrix : Constant  Value=sat.wheel.repartition_matrix_3RW
  If Action Subsystem : Subsystem  TreatAsAtomicUnit=on
  If Action Subsystem1 : Subsystem  TreatAsAtomicUnit=on
  If Action Subsystem2 : Subsystem  TreatAsAtomicUnit=on
  If Action Subsystem3 : Subsystem  TreatAsAtomicUnit=on
  If1 : If  IfExpression=u1 > 0.0068
  If2 : If
  Inertia : Constant  Value=sat.inertia
  Integrative constant Ki : Constant  Value=0.01
  Kd2 : Constant  Commented=on  Value=sat.PID.kd
  Kp : Constant  Commented=on  Value=sat.PID.kp
  Manual Switch : ManualSwitch  CurrentSetting=0
  MatrixMultiply : Product  Multiplication=Matrix(*)
  MatrixMultiply1 : Product  Multiplication=Matrix(*)
  Max of Elements : MinMax  Function=max
  Max of Elements1 : MinMax  Function=max
  Merge : Merge
  Merge1 : Merge
  Min : MinMax  Inputs=2
  Mux : Mux
  Mux1 : Mux  Inputs=2
  Product{1..3,9..10} (5 alike) : Product
  Product4 : Product  Multiplication=Matrix(*)
  Product8 : Product  Multiplication=Matrix(*)
  Proportional constant Kp : Constant  Value=0.5
  Quaternion Inverse : aerolibutil/Quaternion Inverse
  Quaternion Multiplication : aerolibutil/Quaternion Multiplication
  RW1 : Subsystem
  RW2 : Subsystem
  RW3 : Subsystem
  "RW4 " : Subsystem
  Repartition RWA : Constant  Value=sat.wheel.repartition_metrix_4RW_inverse
  Scope1 : Scope  NumInputPorts=2
  Scope2 : Scope
  Scope3 : Scope
  Scope4 : Scope  NumInputPorts=4
  Scope5 : Scope
  Scope6 : Scope  NumInputPorts=2
  Sum : Sum  Inputs=|+-
  kp_mag : Gain  Gain=sat.PID.kpmag
  wheels unused : Constant  Value=[0, 0, 0]
  RW Command : Outport  VectorParamsAs1DForOutWhenUnconnected=off
  Mag Command : Outport  Port=2  VectorParamsAs1DForOutWhenUnconnected=off
  wires:
  No wheels use/1 -> If2/1
  MatrixMultiply/1 -> Abs1/1, Product1/2, Mux1/1  "Torque 4 wheels"
  Command Magnetic moments computation/1(Mag vector command) -> Mag Command/1
  Merge/1 -> Gain/1
  Product8/1 -> If Action Subsystem/1(In1)
  Constant14/1 -> Command Magnetic moments computation/5(h3 (vect))
  Constant12/1 -> Command Magnetic moments computation/3(h1 (vect))
  Constant/1 -> MatrixMultiply1/1
  Manual Switch/1 -> Abs/1, Scope1/2, Average angular velocity/1, Product3/2
  Constant11/1 -> If Action Subsystem3/1(In1)
  If2/2 -> If Action Subsystem/Action
  Max of Elements1/1 -> Divide/2
  Abs1/1 -> Max of Elements1/1
  Average angular velocity/1 -> Scope1/1
  Product10/1 -> Discrete-Time Integrator1/1
  Constant10/1 -> If Action Subsystem2/1(In1)
  Derivative constant Kd/1 -> Product3/1
  Demux/4 -> "RW4 "/1(Mc (scalar))
  Constant6/1 -> Divide/1
  Constant13/1 -> Command Magnetic moments computation/4(h2 (vect))
  Abs/1 -> Max of Elements/1
  Demux/3 -> RW3/1(Mc (scalar))
  Inertia/1 -> Product4/1
  RW3/1(Omega_C (scalar)) -> Mux/3
  Product9/1 -> Scope4/2, Add1/1
  RW2/1(Omega_C (scalar)) -> Mux/2
  Demux/2 -> RW2/1(Mc (scalar))
  RW1/1(Omega_C (scalar)) -> Mux/1
  Demux/1 -> RW1/1(Mc (scalar))
  If Action Subsystem/1(Out1) -> Merge/1
  Mux/1 -> MatrixMultiply1/2, RW Command/1
  If1/2 -> If Action Subsystem3/Action
  Constant7/1 -> Min/2
  If Action Subsystem3/1(Out1) -> Merge1/2
  If Action Subsystem2/1(Out1) -> Merge1/1
  Add1/1 -> Scope4/4, Scope3/1, Product4/2
  Identity matrix/1 -> Product8/1
  Gain1/1 -> Command Magnetic moments computation/1(Command (vect))
  Repartition RWA/1 -> MatrixMultiply/1
  Divide/1 -> Min/1
  Qref_ECI/1 -> Quaternion Multiplication/2
  wheels unused/1 -> If Action Subsystem1/1(In1)
  Max of Elements/1 -> Scope5/1, If1/1
  Merge1/1 -> Scope2/1, Product10/1
  Product4/1 -> Product8/2
  B_IGRF_Body/1 -> Command Magnetic moments computation/2(B_IGRF_body (vect))
  Q_ECI/1 -> Quaternion Inverse/1
  Product2/1 -> Scope4/1, Add1/2
  "RW4 "/1(Omega_C (scalar)) -> Mux/4
  Discrete-Time Integrator1/1 -> Product9/2
  Proportional constant Kp/1 -> Product2/1
  If1/1 -> If Action Subsystem2/Action
  If2/1 -> If Action Subsystem1/Action
  Quaternion Multiplication/1 -> Extract Vect/1(Qr)  "Qr"
  Extract Vect/1(Qvect) -> Product10/2, Product2/2
  Min/1 -> Product1/1
  Integrative constant Ki/1 -> Product9/1
  If Action Subsystem1/1(Out1) -> Merge/2
  Product1/1 -> Mux1/2, Demux/1  "T limit"
  Product3/1 -> Gain2/1
  kp_mag/1 -> Gain1/1
  Quaternion Inverse/1 -> Quaternion Multiplication/1
  MatrixMultiply1/1 -> kp_mag/1
  Gain/1 -> Scope6/1, MatrixMultiply/2  "Torque"
  W_Body/1 -> Sum/1, Manual Switch/1
  W_ref/1 -> Sum/2
  Sum/1 -> Manual Switch/2
  Gain2/1 -> Add1/3, Scope4/3
  Mux1/1 -> Scope6/2

== system IonSatSimulationE/Attitude Controller/RW4 ==
  note: Entrées:
      | - Moment de commande (déjà projeté sur l'axe de la roue...)
      | Sorties:
      | - Omega de commande à appliquer
  Mc (scalar) : Inport
  Divide : Product  Inputs=*/
  Saturation_speed : Saturate  UpperLimit=sat.wheel.max_speed  LowerLimit=- sat.wheel.max_speed
  Torque_sat : Saturate  UpperLimit=sat.wheel.max_torque  LowerLimit=- sat.wheel.max_torque
  Wheel Inertia : Constant  Value=sat.wheel.max_sigma/sat.wheel.max_speed
  Omega_C (scalar) : Outport
  wires:
  Mc (scalar)/1 -> Torque_sat/1
  Wheel Inertia/1 -> Divide/2
  Divide/1 -> ?  "dw/dt"
  ? -> Saturation_speed/1
  Torque_sat/1 -> Divide/1  "Torque (scal)"
  Saturation_speed/1 -> Omega_C (scalar)/1
